simulink model "testerzagrozen"  (R2022b)
settings: Solver=VariableStepAuto  StartTime=0.0  StopTime=10  RelTol=1e-3
values from neighbouring files (symbols this model uses):
  ACCtime = 0    [dane.m]    (also in szybkiwykres.m; wykresownikfinalny.m)
libraries: simulink x4
settings Model: Creator=48519  LastModifiedBy=48519
settings ModelReferenceCC: EnableRefExpFcnMdlSchedulingChecks=on

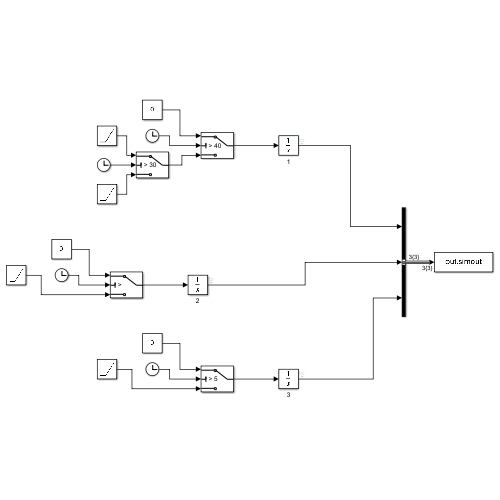
[thumbnail: Simulink's stored preview of the top-level diagram]
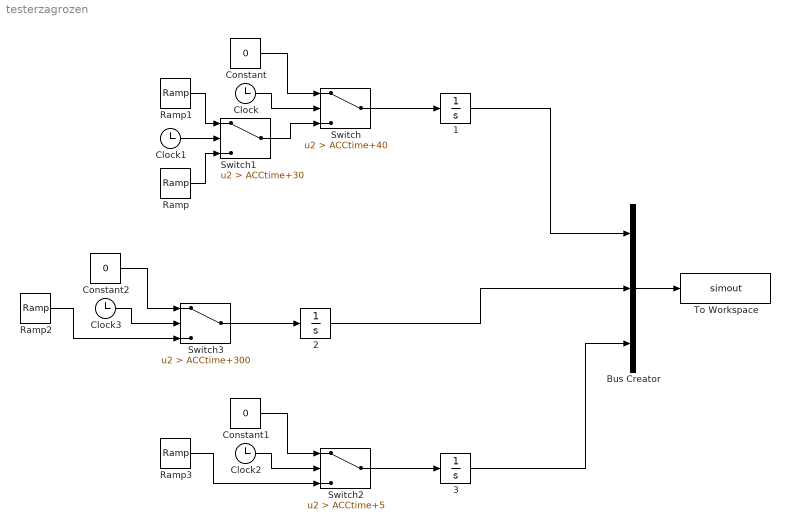
== system testerzagrozen ==
  1 : Integrator
  2 : Integrator
  3 : Integrator
  Bus Creator : BusCreator  Inputs=3
  Clock{,1..3} (4 alike) : Clock
  Constant : Constant  Value=0
  Constant1 : Constant  Value=0
  Constant2 : Constant  Value=0
  Ramp : simulink/Sources/Ramp  slope=-0.07/450  start=ACCtime  InitialOutput=0
  Ramp1 : simulink/Sources/Ramp  slope=0.07/50  start=ACCtime+30  InitialOutput=0
  Ramp2 : simulink/Sources/Ramp  slope=-(0.05)/(300*300/2)  start=ACCtime  InitialOutput=0
  Ramp3 : simulink/Sources/Ramp  slope=-0.6/25  start=ACCtime  InitialOutput=0
  Switch : Switch  Criteria=u2 > Threshold  Threshold=ACCtime+40  SaturateOnIntegerOverflow=off  InputSameDT=off
  Switch1 : Switch  Criteria=u2 > Threshold  Threshold=ACCtime+30  SaturateOnIntegerOverflow=off  InputSameDT=off
  Switch2 : Switch  Criteria=u2 > Threshold  Threshold=ACCtime+5  SaturateOnIntegerOverflow=off  InputSameDT=off
  Switch3 : Switch  Criteria=u2 > Threshold  Threshold=ACCtime+300  SaturateOnIntegerOverflow=off  InputSameDT=off
  To Workspace : ToWorkspace  VariableName=simout  SaveFormat=Timeseries  SampleTime=-1
  wires:
  Ramp1/1 -> Switch1/1
  Switch/1 -> 1/1
  Clock/1 -> Switch/2
  Constant/1 -> Switch/1
  Clock1/1 -> Switch1/2
  Ramp/1 -> Switch1/3
  Switch1/1 -> Switch/3
  Switch2/1 -> 3/1
  Ramp3/1 -> Switch2/3
  Constant1/1 -> Switch2/1
  Clock2/1 -> Switch2/2
  Bus Creator/1 -> To Workspace/1
  3/1 -> Bus Creator/3
  1/1 -> Bus Creator/1
  2/1 -> Bus Creator/2
  Ramp2/1 -> Switch3/3
  Clock3/1 -> Switch3/2
  Constant2/1 -> Switch3/1
  Switch3/1 -> 2/1
